simulink model "LQR_discrete_hkn"  (R2018b)
settings: Solver=ode45  StartTime=0.0  StopTime=T_sim  RelTol=1e-3  EnableMultiTasking=on
values from neighbouring files (symbols this model uses):
  Kdlqr_simulink = Kdlqr    [Q7.m]
  set_point = [5000;10;1000;0]    [Q7.m]
  sys_discrete = c2d(sys, Ts)    [Q7.m]
  Ts = 0.25    [Q7.m]
  u_max_simulink = u_max    (= 0.262)    [Q7.m]
  u_min_simulink = u_min    (= -0.262)    [Q7.m]
  x0 = [0;0;0;10]    [Q7.m]
settings Model: Creator=lele  LastModifiedBy=HknHtc
settings DataIOCC: LimitDataPoints=on  SaveFormat=Array
settings OptimizationCC: LifeSpan=inf
settings DebuggingCC: SolverPrmCheckMsg=warning  SFUnexpectedBacktrackingDiag=warning  SFNoUnconditionalDefaultTransitionDiag=warning  SFExecutionAtInitializationDiag=none
settings HardwareCC: ProdBitPerPointer=32  ProdBitPerSizeT=32  ProdBitPerPtrDiffT=32  ProdLargestAtomicFloat=None  ProdIntDivRoundTo=Undefined  ProdEndianess=Unspecified  ProdWordSize=32  ProdHWDeviceType=32-bit Generic
settings ModelReferenceCC: PropagateSignalLabelsOutOfModel=off
settings SFSimCC: SimUseLocalCustomCode=off
settings RTWCC: RTWUseLocalCustomCode=off
settings CodeAppCC: StateflowObjectComments=on
settings GRTTargetCC: TargetLangStandard=C89/C90 (ANSI)  GeneratePreprocessorConditionals=Disable all
settings ConfigComp: CovMetricSettings=dw  CovHtmlReporting=on  CovSaveCumulativeToWorkspaceVar=on  CovSaveSingleToWorkspaceVar=on  CovExternalEMLEnable=off  CovSFcnEnable=off

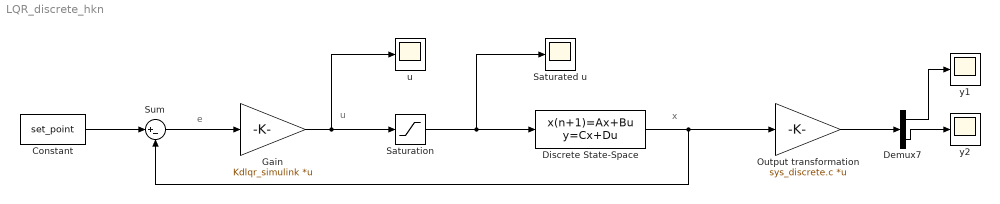
== system LQR_discrete_hkn ==
  note: x
  note: u
  note: e
  Constant : Constant  Value=set_point
  Demux7 : Demux  Outputs=2
  Discrete State-Space : DiscreteStateSpace  A=sys_discrete.a  B=sys_discrete.b  C=eye(4)  D=zeros(4, 1)  InitialCondition=x0  SampleTime=Ts
  Gain : Gain  Gain=Kdlqr_simulink  Multiplication=Matrix(K*u)
  Output transformation : Gain  Gain=sys_discrete.c  Multiplication=Matrix(K*u)
  Saturated u : Scope
  Saturation : Saturate  UpperLimit=u_max_simulink  LowerLimit=u_min_simulink
  Sum : Sum  Inputs=|+-
  u : Scope
  y1 : Scope
  y2 : Scope
  wires:
  Constant/1 -> Sum/1
  Sum/1 -> Gain/1
  Gain/1 -> u/1, Saturation/1
  Saturation/1 -> Discrete State-Space/1, Saturated u/1
  Output transformation/1 -> Demux7/1
  Demux7/1 -> y1/1
  Demux7/2 -> y2/1
  Discrete State-Space/1 -> Output transformation/1, Sum/2
